simulink subsystem "PvtSubSys_PLAN_AP"  (R2020b)
settings: Solver=VariableStepAuto  StartTime=0.0  StopTime=10.0  RelTol=1e-3
undefined symbols (not defined in the file or in its folder): C_LongCtrl_0_Single, C_LongCtrl_0_Uint8, C_LongCtrl_Mph2Kph, magnitude, P_LongCtrl_accelTargAbsThrd, P_LongCtrl_AddVelAccelChange, P_LongCtrl_AddVelAccelThrd, P_LongCtrl_AddVelDistDesThrd, P_LongCtrl_AddVelEnable, P_LongCtrl_AddVelRefMsThrd, P_LongCtrl_ALaLowerChar, P_LongCtrl_ALaUpperCharEco, P_LongCtrl_ALaUpperCharNormal, P_LongCtrl_ALaUpperCharSport, P_LongCtrl_ALCAccLimitByDangerXAxis, P_LongCtrl_ALCAccLimitByDangerYAxis, P_LongCtrl_ALvAcceleLowerChar, P_LongCtrl_ALvAcceleUpperCharEco, P_LongCtrl_ALvAcceleUpperCharNormal, P_LongCtrl_ALvAcceleUpperCharSport, P_LongCtrl_CCaccelCCNeg2PosJerk, P_LongCtrl_CCaccelCCPosJerk, P_LongCtrl_CCaccelLowerIsLaneChange, P_LongCtrl_CCaccelMaxLCActive, P_LongCtrl_CCaccelMinECOAL, P_LongCtrl_CCaccelMinFastDecel, P_LongCtrl_CCaccelMinNoFastDecel, P_LongCtrl_CCaccelMinNormAL, P_LongCtrl_CCaccelMinSportAL, P_LongCtrl_CCaccelUpperCC, P_LongCtrl_CCaccelUpperCCSafeStop, P_LongCtrl_CCaMinNegAcceleLowerBand, P_LongCtrl_CCaMinNegAcceleUpperBand, P_LongCtrl_CCaMinPosAcceleLowerBand, P_LongCtrl_CCaMinPosAcceleUpperBand, P_LongCtrl_CCbECO, P_LongCtrl_CCbNorm, P_LongCtrl_CCbSport, P_LongCtrl_CCcoefESPSpd2IPSpd1, P_LongCtrl_CCcoefESPSpd2IPSpd2, P_LongCtrl_CCdecelCCJerk, P_LongCtrl_CCdecelCCJerkNegVLCInternalAcc, P_LongCtrl_CCfacNegAcceleLowerBand, P_LongCtrl_CCfacNegAcceleUpperBand, P_LongCtrl_CCfacPosAcceleLowerBand, P_LongCtrl_CCfacPosAcceleUpperBand, P_LongCtrl_CCkECO, P_LongCtrl_CCkNorm, P_LongCtrl_CCkSport, P_LongCtrl_CCLCIncSetSpdAdd, P_LongCtrl_CCLCIncSetSpdAddCntStartValue, P_LongCtrl_CCResumeDelayDeltaVel, P_LongCtrl_CCtAcceleTimeNeg, P_LongCtrl_CCtAcceleTimeNegCorrXAxis, P_LongCtrl_CCtAcceleTimeNegCorrYAxis, P_LongCtrl_CCtAcceleTimePos, P_LongCtrl_CCtAcceleTimePosCorrXAxis, P_LongCtrl_CCtAcceleTimePosCorrYAxis, P_LongCtrl_CCtStepVelPlan, P_LongCtrl_CCtTotVelPlan ... (+150)
libraries: simulink x62, TrueDurationTime x1
(part 7 of 7)

== matlab function PvtSubSys_PLAN_AP/AP/AP/FollowCtrl/VelTargPlanTerminateCalc/VelTarAbsTerminateCalc ==
  data: vf input single; af input single; vterminate output single size=[20,1]
function vterminate   = fcn(vf,af)
vterminate=single(zeros(20,1));
 for i=1:20
     t=single(0.5)+single(i)-single(1);
     vterminate(i,:) = max(single(0),vf+af*t);
     if vterminate(i,:)<0.1
         vterminate(i,:)=single(0);
     end
 end

== stateflow chart PvtSubSys_PLAN_AP/AP/AP/FollowCtrl/AccelTargAbsEnableJudge/AccelTargAbsEnableJudge ==
  (default) -> (junction 122)
  (junction 122) -> (junction 123) [order 1] : [IDP0(1)==IDP0(2)]
  (junction 122) -> (junction 127) [order 2] : {accelTargAbsK1=accelTargAbsFilt;}
  (junction 123) -> (junction 125)
  (junction 125) -> (junction 127)
  (junction 127) -> (junction 1)
  (junction 1) -> (junction 3) [order 1] : [(accelTargAbsFilt<C_accelTargAbsEnableNegMax)||...
      |  ((distTargRel<C_distTargRelEnableAccelTargAbsThres)&&(accelTargAbsFilt<C_accelTargAbsEnableRangeMax))]
  (junction 1) -> (junction 10) [order 2]
  (junction 3) -> (junction 7) : {accelTargAbsEnableNegFlag=true;}
  (junction 7) -> (junction 10)
  (junction 10) -> (junction 13)
  (junction 13) -> (junction 30) [order 1] : [(accelTargAbsEnableNegFlag==true)&&...
      | (accelTargAbsFilt<C_accelTargAbsExitNegMin)]
  (junction 13) -> (junction 43) [order 2]
  (junction 30) -> (junction 32)
  (junction 32) -> (junction 34) [order 1] : [accelTargAbsK1>=accelTargAbsFilt]
  (junction 32) -> (junction 38) [order 2] : {accelTargAbs=min(accelTargAbsK1+C_accelTargAbsEnablePosJerk*tCycle,accelTargAbsFilt);}
  (junction 34) -> (junction 36) : {accelTargAbs=max(accelTargAbsK1+C_accelTargAbsEnableNegJerk*tCycle,accelTargAbsFilt);}
  (junction 38) -> (junction 43)
  (junction 36) -> (junction 38)
  (junction 43) -> (junction 64)
  (junction 64) -> (junction 58) [order 1] : [(accelTargAbsEnableNegFlag==true&&...
      |  accelTargAbsFilt>C_accelTargAbsExitNegMin)]
  (junction 64) -> (junction 62) [order 2]
  (junction 58) -> (junction 60) : {accelTargAbs=min(accelTargAbsK1+C_accelTargAbsEnablePosJerk*tCycle,single(0));}
  (junction 60) -> (junction 66) [order 1] : [accelTargAbs==0]
  (junction 60) -> (junction 70) [order 2]
  (junction 66) -> (junction 68) : {accelTargAbsEnableNegFlag=false;}
  (junction 70) -> (junction 62)
  (junction 68) -> (junction 70)
  (junction 62) -> (junction 117) : {accelTargAbsK1=accelTargAbs;}
  data: IDP0 input; distTargRel input; accelTargAbsFilt input single; tCycle input single; C_accelTargAbsEnableNegMax input single; accelTargAbs output single =single(0); C_accelTargAbsEnableNegJerk input single; C_accelTargAbsExitNegMin input single; accelTargAbsEnableNegFlag local boolean =false; C_accelTargAbsEnablePosJerk input single; C_distTargRelEnableAccelTargAbsThres input; C_accelTargAbsEnableRangeMax input; accelTargAbsK1 local single

== stateflow chart PvtSubSys_PLAN_AP/AP/AP/FollowCtrl/AccelTargFilter/accelTargAbsFilter ==
  state tFiltP0 = tFiltP0Calc(diffAccelCur2K1P0) [function]
  (default) -> (junction 1)
  (junction 1) -> (junction 3) [order 1] : [IDP0(1)~=0]
  (junction 1) -> (junction 7) [order 2] : {accelTargAbsFiltP0=single(0);}
  (junction 3) -> (junction 5) : {accelTargAbsFiltP0K1Set=accelTargAbsP0;}
  (junction 5) -> (junction 11) [order 1] : [IDP0(1)==IDP0(2)]
  (junction 5) -> (junction 17) [order 2]
  (junction 11) -> (junction 15) : {accelTargAbsFiltP0K1Set=accelTargAbsFiltP0K1;}
  (junction 17) -> (junction 19) [order 1] : [IDP0(1)==IDP2(2)]
  (junction 17) -> (junction 23) [order 2]
  (junction 19) -> (junction 21) : {accelTargAbsFiltP0K1Set=accelTargAbsFiltP2K1;}
  (junction 23) -> (junction 26) [order 1] : [IDP0(1)==IDP3(2)]
  (junction 23) -> (junction 30) [order 2]
  (junction 26) -> (junction 28) : {accelTargAbsFiltP0K1Set=accelTargAbsFiltP3K1;}
  (junction 28) -> (junction 30)
  (junction 21) -> (junction 28)
  (junction 15) -> (junction 21)
  (junction 30) -> (junction 36) : {tFiltP0=single(0.5);
      |  diffAccelCur2K1P0=accelTargAbsP0-accelTargAbsFiltP0K1Set;}
  (junction 36) -> (junction 38) [order 1] : [diffAccelCur2K1P0<0]
  (junction 36) -> (junction 42) [order 2]
  (junction 38) -> (junction 40) : {tFiltP0 = tFiltP0Calc(diffAccelCur2K1P0);}
  (junction 40) -> (junction 42)
  (junction 42) -> (junction 48) : {accelTargAbsFiltP0=(accelTargAbsP0-accelTargAbsFiltP0K1Set)*single(0.05)/tFiltP0+accelTargAbsFiltP0K1Set;}
  (junction 48) -> (junction 7)
  (junction 7) -> (junction 51)
  (junction 51) -> (junction 53) [order 1] : [IDP2(1)~=0]
  (junction 51) -> (junction 57) [order 2] : {accelTargAbsFiltP2=single(0);}
  (junction 53) -> (junction 55) : {accelTargAbsFiltP2=(accelTargAbsP2-accelTargAbsFiltP2K1)*single(0.05)/single(0.5)+accelTargAbsFiltP2K1;}
  (junction 55) -> (junction 57)
  (junction 57) -> (junction 60)
  (junction 60) -> (junction 65) [order 1] : [IDP3(1)~=0]
  (junction 60) -> (junction 66) [order 2] : {accelTargAbsFiltP3=single(0);}
  (junction 65) -> (junction 67) : {accelTargAbsFiltP3=(accelTargAbsP3-accelTargAbsFiltP3K1)*single(0.05)/single(0.5)+accelTargAbsFiltP3K1;}
  (junction 67) -> (junction 66)
  (junction 66) -> (junction 69) : {accelTargAbsFiltP0K1=accelTargAbsFiltP0;
      |  accelTargAbsFiltP2K1=accelTargAbsFiltP2;
      |  accelTargAbsFiltP3K1=accelTargAbsFiltP3;}
  data: diffAccelCur2K1P0 function_input single size=1; tFiltP0 function_output; IDP0 input; IDP2 input; IDP3 input; accelTargAbsP0 input; accelTargAbsFiltP0K1Set local; accelTargAbsP2 input; accelTargAbsP3 input; accelTargAbsFiltP0 output; accelTargAbsFiltP2 local; accelTargAbsFiltP0K1 local; accelTargAbsFiltP2K1 local; accelTargAbsFiltP3 local; accelTargAbsFiltP3K1 local; diffAccelCur2K1P0 local; tFiltP0 local

== stateflow chart PvtSubSys_PLAN_AP/AP/AP/FollowCtrl/DecelToStopCtrl/DecelToStopCtrl/DecelToStopCtrl ==
  (default) -> (junction 1)
  (junction 1) -> (junction 3) [order 1] : [(distTargRel<P_LongCtrl_distThresEnableStop)&&...
      |  (accelTargAbs<P_LongCtrl_accelTargThresEnableStop)&&...
      |  (velSubj<(P_LongCtrl_velSubjThresEnableStop+velSubjThresEnableStopAdd))&&...
      |  (FollowAccelDes<accelFollowDesThresEnableStop)&&...
      |  (DrvOFF_Req==false)]
  (junction 3) -> (junction 90) [order 1] : [(FollowAccelDes>P_LongCtrl_AddVelAccelThrd)&&(distTargRel>(distDesCur+P_LongCtrl_AddVelDistDesThrd))&&(velSubj<P_LongCtrl_AddVelRefMsThrd)&&(P_LongCtrl_AddVelEnable==1)]
  (junction 1) -> (junction 13) [order 2] : {FollowAccel=FollowAccelDes;
      |  counter =single(0);
      |  accelForce=single(0);
      |  ForceStop=false;}
  (junction 3) -> (junction 22) [order 2] : {FollowAccel=min(FollowAccelDes,P_LongCtrl_accelStopMax);
      |  distDesCurCorr=distDesCur+P_LongCtrl_FollowDistDesAddForceStop;}
  (junction 90) -> (junction 92) : {FollowAccel = P_LongCtrl_AddVelAccelChange;
      |  counter =single(0);
      |  accelForce=single(0);
      |  ForceStop=false;}
  (junction 22) -> (junction 23) [order 1] : [((velSubj<velSubjThresForceStop)&&...
      |  (distTargRel<distDesCurCorr)&&...
      |  (accelTargAbs<P_LongCtrl_accelTargThresForceStop))||...
      | (((velTargAbs<P_LongCtrl_velTarAbsThresForceStop)||(ObjMovingStateP0==4)||(ObjMovingStateP0==3))&&(velSubj<velSubjThresForceStopStationaryTarget)&&(distTargRel<distDesCurCorr))]
  (junction 22) -> (junction 27) [order 2] : {counter =single(0);
      |  accelForce=single(0);
      |  ForceStop=false;}
  (junction 23) -> (junction 38) : {ForceStop=true;}
  (junction 38) -> (junction 40) [order 1] : [(ACCModeStsK1==3&&(ACCModeSts==6||ACCModeSts==9))||...
      |  (accelForceClear==true)]
  (junction 40) -> (junction 49)
  (junction 38) -> (junction 59) [order 2]
  (junction 49) -> (junction 74) [order 1] : [accelForce<0]
  (junction 49) -> (junction 54) [order 2] : {accelForceClear=false;}
  (junction 74) -> (junction 50)
  (junction 59) -> (junction 61) [order 1] : [accelForceClear==false&&(ACCModeSts==6||ACCModeSts==9)]
  (junction 59) -> (junction 65) [order 2] : {counter = min(single(300),counter + single(1));
      |  accelForce=max(accelForceMin,jerkForceStop*counter);}
  (junction 61) -> (junction 63) : {counter =single(0);
      |  accelForce=single(0);}
  (junction 50) -> (junction 69) [order 1] : [(ACCModeStsK1==6||ACCModeStsK1==9)&&...
      |  (ACCModeSts~=6&&ACCModeSts~=9)]
  (junction 50) -> (junction 68) [order 2] : {counter = max(single(0),counter - single(1));
      |  accelForce=max(accelForceMin,jerkForceStop*counter);
      |  accelForceClear=true;}
  (junction 69) -> (junction 71) : {counter =single(0);
      |  accelForce=single(0);}
  (junction 71) -> (junction 68)
  (junction 68) -> (junction 52)
  (junction 52) -> (junction 54)
  (junction 54) -> (junction 42)
  (junction 63) -> (junction 65)
  (junction 65) -> (junction 44)
  (junction 42) -> (junction 44)
  (junction 44) -> (junction 25)
  (junction 25) -> (junction 27)
  (junction 27) -> (junction 11) : {FollowAccel=FollowAccel+accelForce;}
  (junction 11) -> (junction 13)
  (junction 92) -> (junction 11)
  (junction 13) -> (junction 16) : {ACCModeStsK1=ACCModeSts;}
  data: accelTargAbs input single; velSubj input single; FollowAccelDes input single; distDesCur input; velTargAbs input; ACCModeSts input; DrvOFF_Req input; distTargRel input single; accelFollowDesThresEnableStop input single; velSubjThresEnableStopAdd input; velSubjThresForceStopStationaryTarget input; velSubjThresForceStop input; jerkForceStop input; accelForceMin input single; P_LongCtrl_distThresEnableStop input single; P_LongCtrl_velSubjThresEnableStop input single; P_LongCtrl_accelTargThresEnableStop input single; P_LongCtrl_accelStopMax input single; FollowAccel output single; P_LongCtrl_accelTargThresForceStop input; counter local =single(0); accelForce local; ACCModeStsK1 local =uint8(0); accelForceClear local =false; distDesCurCorr local; P_LongCtrl_velTarAbsThresForceStop input; ForceStop output =false; P_LongCtrl_FollowDistDesAddForceStop parameter; ObjMovingStateP0 input; P_LongCtrl_AddVelAccelThrd input; P_LongCtrl_AddVelDistDesThrd input; P_LongCtrl_AddVelRefMsThrd input; P_LongCtrl_AddVelEnable input; P_LongCtrl_AddVelAccelChange input

== matlab function PvtSubSys_PLAN_AP/AP/AP/FollowCtrl/DistRelPlanTerminateCalc/DistRelPlanTerminateCalc2 ==
  data: R input single; distDesPlanCorr input single; velTargAbsPlanTerminate input; vf input single; af input single; Dterminate output single size=[20,1]; DterminateMin input; tTargStop output; distTargPlan output; velSubj input
function [Dterminate,tTargStop,distTargPlan]  = fcn(R,distDesPlanCorr,velTargAbsPlanTerminate,vf,af,DterminateMin,velSubj)
Dterminate=single(zeros(20,1));
if af<0
   tTargStop=(-vf/min(single(-0.01),af)); 
else
   tTargStop=single(100); 
end
% tTargStop=(-vf/min(single(-0.01),af));
jTargStop=fix(tTargStop+single(0.5));
if (jTargStop>=0)&&(jTargStop<=19)
    distTargPlan=vf*tTargStop +single(0.5)*af*tTargStop^2;
else
    distTargPlan=single(0);
end

for i=1:20
    t=single(0.5+i-1);
    if velSubj<5
           DterminateMinCalc=(velSubj-velTargAbsPlanTerminate(i))^2/single(6);
        else
           DterminateMinCalc=single(0); 
    end
    DterminateMin=max(DterminateMin,DterminateMinCalc);
    if i<=jTargStop
        Dterminate(i,:) = max(DterminateMin,R+ vf*t +single(0.5)*af*t^2 -distDesPlanCorr(i,:));
    else
        Dterminate(i,:) = max(DterminateMin,R+ distTargPlan -distDesPlanCorr(i,:));
    end
end

== stateflow chart PvtSubSys_PLAN_AP/AP/AP/FollowCtrl/FollowBandJerkCalc/DecelFollowJerkCalc/OverrideJerk ==
  state lowerJerkOverride = lowerJerkOverrideCalc(VlcInternalAccK1) [function]
  (default) -> (junction 1)
  (junction 1) -> (junction 3) [order 1] : [ACCModeSts==5]
  (junction 1) -> (junction 29) [order 2]
  (junction 3) -> (junction 5) : {lowerJerkOverride = lowerJerkOverrideCalc(VlcInternalAccK1);}
  (junction 29) -> (junction 30) [order 1] : [VlcInternalAccK1>0]
  (junction 29) -> (junction 34) [order 2] : {lowerJerkOverride=single(0);}
  (junction 30) -> (junction 32) : {lowerJerkOverride=min(single(0),lowerJerkOverride+dtJerk*tCycle);}
  (junction 32) -> (junction 34)
  (junction 34) -> (junction 7)
  (junction 5) -> (junction 7)
  (junction 7) -> (junction 19)
  (junction 19) -> (junction 38) [order 1] : [ACCModeSts~=3&&ACCModeSts~=4&&ACCModeSts~=5&&ACCModeSts~=6&&ACCModeSts~=9]
  (junction 19) -> (junction 42) [order 2]
  (junction 38) -> (junction 40) : {lowerJerkOverride=single(0);}
  (junction 40) -> (junction 42)
  (junction 42) -> (junction 45)
  data: VlcInternalAccK1 function_input single size=1; lowerJerkOverride function_output; ACCModeSts input; dtJerk input; tCycle input; lowerJerkOverride output single =single(0); VlcInternalAccK1 input single

== stateflow chart PvtSubSys_PLAN_AP/AP/AP/FollowCtrl/PlausibilityCheck/StandstillOverride ==
  (default) -> (junction 1)
  (junction 1) -> (junction 3) [order 1] : [(velTargAbs<P_LongCtrl_FollowvelTargAbsMaxJudgeStationaryTarget)&&(distTargRel<P_LongCtrl_FollowdistRelMaxJudgeStationaryTarget)]
  (junction 1) -> (junction 9) [order 2] : {targetIsStopped=false;}
  (junction 3) -> (junction 7) : {targetIsStopped=true;}
  (junction 7) -> (junction 9)
  (junction 9) -> (junction 13)
  (junction 13) -> (junction 15) [order 1] : [ACCModeK1==5&&ACCMode==3]
  (junction 13) -> (junction 19) [order 2]
  (junction 15) -> (junction 17) : {ACCModeStateFullFill=true;}
  (junction 19) -> (junction 24) [order 1] : [(ACCModeK1==3&&ACCMode~=3)||...
      |  (targetIsStopped==false)]
  (junction 19) -> (junction 28) [order 2]
  (junction 24) -> (junction 26) : {ACCModeStateFullFill=false;}
  (junction 26) -> (junction 28)
  (junction 28) -> (junction 31)
  (junction 17) -> (junction 31)
  (junction 31) -> (junction 36)
  (junction 36) -> (junction 38) [order 1] : [ACCModeStateFullFill==true&&targetIsStopped==true]
  (junction 36) -> (junction 42) [order 2] : {coefStandstillOverride=single(1);
      |  standstillOverrideCondition=false;}
  (junction 38) -> (junction 50) : {standstillOverrideCondition=true;}
  (junction 50) -> (junction 51) [order 1] : [FollowAccele_Plau<0.5]
  (junction 50) -> (junction 55) [order 2]
  (junction 51) -> (junction 53) : {coefStandstillOverride=P_LongCtrl_FollowcoefAccelStandstillOverride;}
  (junction 53) -> (junction 55)
  (junction 55) -> (junction 40)
  (junction 40) -> (junction 42)
  (junction 42) -> (junction 45) : {ACCModeK1=ACCMode;}
  data: standstillOverrideCondition output boolean; FollowAccele_Plau input; velTargAbs input; distTargRel input; targetIsStopped local; ACCModeStateFullFill local =false; ACCModeK1 local uint8 =uint8(0); ACCMode input uint8; coefStandstillOverride output; P_LongCtrl_FollowvelTargAbsMaxJudgeStationaryTarget parameter; P_LongCtrl_FollowdistRelMaxJudgeStationaryTarget parameter; P_LongCtrl_FollowcoefAccelStandstillOverride parameter

== stateflow chart PvtSubSys_PLAN_AP/AP/AP/FollowCtrl/SlopeStartupAssist/Chart ==
  (default) -> (junction 1)
  (junction 1) -> (junction 3) [order 1] : [slopeStartupAssist==true]
  (junction 1) -> (junction 7) [order 2] : {accelSlopeAssist=max(single(0),accelSlopeAssist-accelSlopeAssistStep*single(3));}
  (junction 3) -> (junction 5) : {accelSlopeAssist=min(accelSlopeAssistMax,accelSlopeAssist+accelSlopeAssistStep);}
  (junction 5) -> (junction 7)
  (junction 7) -> (junction 12)
  data: slopeStartupAssist input; accelSlopeAssist output =single(0); accelSlopeAssistMax input; accelSlopeAssistStep input

== stateflow chart PvtSubSys_PLAN_AP/AP/AP/FollowCtrl/SlopeStartupAssist/Chart1 ==
  state coefVelTargRel2Accel = coefVelTargRel2AccelCalc(velTargRel) [function]
  state coefDistTargRel2Accel = coefDistTargRel2AccelCalc(distTargRel,distDesCur) [function]
  (default) -> (junction 49)
  (junction 49) -> (junction 52) [order 1] : [((ACCModeStsK1==6||ACCModeStsK1==9)&&ACCModeSts==3)||...
      | ((ACCModeStsK1==5)&&(ACCModeSts==3)&&(velSubj<1))]
  (junction 49) -> (junction 56) [order 2] : {tStartUpEnable=max(single(0),tStartUpEnable-tCycle);}
  (junction 52) -> (junction 54) : {tStartUpEnable=P_LongCtrl_FollowtStartUpAssistEnableMax;}
  (junction 54) -> (junction 56)
  (junction 56) -> (junction 1)
  (junction 1) -> (junction 3) [order 1] : [accelFollowAfterLaneChangeSupress>P_LongCtrl_FollowAccelDesThresStartUpAssistEnable&&...
      |  velTargAbs>P_LongCtrl_FollowVelTargAbsThresStartUpAssistEnable&&...
      |  P_LongCtrl_FollowStartUpAssist==true]
  (junction 1) -> (junction 7) [order 2] : {coefVelDist2Accel=single(1);}
  (junction 3) -> (junction 5)
  (junction 5) -> (junction 10) [order 1] : [(velSubj<P_LongCtrl_FollowVelSubjThresStartUpAssistEnable)&&(velTargRel>0||distTargRel>distDesCur)&&(tStartUpEnable>0)]
  (junction 5) -> (junction 14) [order 2]
  (junction 10) -> (junction 12) : {coefVelTargRel2Accel = coefVelTargRel2AccelCalc(velTargRel);
      |  coefDistTargRel2Accel = coefDistTargRel2AccelCalc(distTargRel,distDesCur);
      |  coefVelDist2Accel=min(single(2),coefVelTargRel2Accel*coefDistTargRel2Accel);}
  (junction 14) -> (junction 33) [order 1] : [coefVelDist2Accel>1]
  (junction 14) -> (junction 37) [order 2] : {coefVelDist2Accel=single(1);}
  (junction 33) -> (junction 35) : {coefVelDist2Accel=max(single(1),coefVelDist2Accel*P_LongCtrl_FollowCoefStartUpAssistFadeOut);}
  (junction 35) -> (junction 37)
  (junction 12) -> (junction 35)
  (junction 37) -> (junction 41)
  (junction 41) -> (junction 7)
  (junction 7) -> (junction 44) : {ACCModeStsK1=ACCModeSts;}
  data: velTargRel function_input single size=1; coefVelTargRel2Accel function_output; distTargRel function_input single size=1; distDesCur function_input single size=1; coefDistTargRel2Accel function_output; velSubj input; accelFollowAfterLaneChangeSupress input; velTargAbs input; distDesCur input; distTargRel input; velTargRel input; coefDistTargRel2Accel local; coefVelTargRel2Accel local; P_LongCtrl_FollowStartUpAssist parameter; coefVelDist2Accel output =single(1); ACCModeSts input; ACCModeStsK1 local =uint8(0); tCycle input; tStartUpEnable local =single(0); P_LongCtrl_FollowtStartUpAssistEnableMax parameter; P_LongCtrl_FollowAccelDesThresStartUpAssistEnable parameter; P_LongCtrl_FollowVelTargAbsThresStartUpAssistEnable parameter; P_LongCtrl_FollowVelSubjThresStartUpAssistEnable parameter; P_LongCtrl_FollowCoefStartUpAssistFadeOut parameter
